simulink model "PM_fnc100a_DevHarness"  (R2022a)
settings: Solver=FixedStepDiscrete  StartTime=1  StopTime=inf  FixedStep=0.01  RelTol=1e-3
values from neighbouring files (symbols this model uses):
  rate_ms = 10    [PM_fnc1000_tc01_iter01_testsignal_builder.m]    (also in PM_fnc21_tc01_iter01_testsignal_builder.m; PM_fnc22_tc01_iter01_testsignal_builder.m)
undefined symbols (not defined in the file or in its folder): cal_abs_ampslimit_hyst_A, cal_abs_ampslimit_thresh_A, cal_cell_heat2cool_factor, cal_chg_falling_slew_rate, cal_chg_PL1_ini, cal_chg_rising_slew_rate, cal_ChgPL1_expiry_dur_thresh_ms, cal_ChgPL2_expiry_dur_thresh_ms, cal_dchg_falling_slew_rate, cal_dchg_PL1_ini, cal_dchg_rising_slew_rate, cal_DchgPL1_expiry_dur_thresh_ms, cal_DchgPL2_expiry_dur_thresh_ms, cal_table_cell_soc_percent, cal_table_cell_temp_degC, cal_table_DchgPL1_10s_limits_xtempysoc, cal_table_DchgPL1_60s_limits_xtempysoc, cal_table_DchgPL1_cont_limits_xtempysoc, cal_table_XLoad_amps_A, cal_table_XLoad_dur_ms
libraries: PM_lib x6
settings Model: PacingRate=1.600000  Creator=306427  LastModifiedBy=306427
settings SolverCC: ZeroCrossAlgorithm=Adaptive

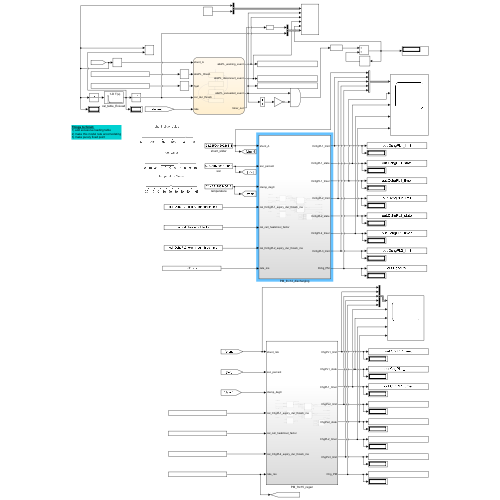
[thumbnail: Simulink's stored preview of the top-level diagram]
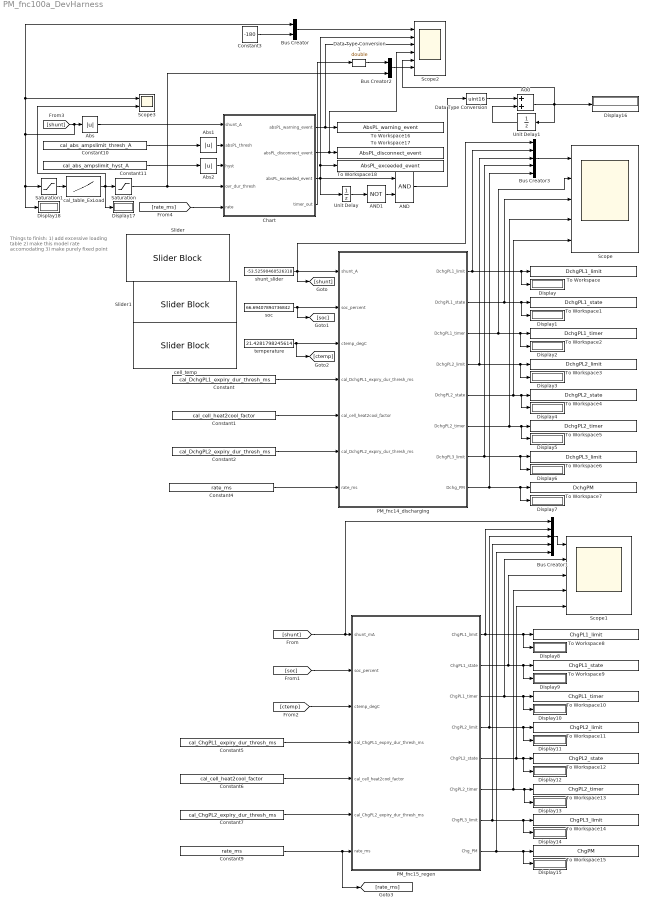
== system PM_fnc100a_DevHarness ==
  note: Things to finish:
      | 1) add excessive loading table
      | 2) make this model rate accomodating
      | 3) make purely fixed point
  AND : Logic  IconShape=distinctive  AllPortsSameDT=off  OutDataTypeStr=boolean
  AND1 : Logic  Operator=NOT  IconShape=distinctive  AllPortsSameDT=off  OutDataTypeStr=boolean
  Abs : Abs  SaturateOnIntegerOverflow=off
  Abs1 : Abs  SaturateOnIntegerOverflow=off
  Abs2 : Abs  SaturateOnIntegerOverflow=off
  Add : Sum
  Bus Creator : BusCreator  Inputs=2
  Bus Creator1 : BusCreator  Inputs=5
  Bus Creator2 : BusCreator  Inputs=2
  Bus Creator3 : BusCreator  Inputs=5
  Chart : Stateflow chart  TreatAsAtomicUnit=on
  Constant : Constant  Value=cal_DchgPL1_expiry_dur_thresh_ms
  Constant1 : Constant  Value=cal_cell_heat2cool_factor
  Constant10 : Constant  Value=cal_abs_ampslimit_thresh_A
  Constant11 : Constant  Value=cal_abs_ampslimit_hyst_A
  Constant2 : Constant  Value=cal_DchgPL2_expiry_dur_thresh_ms
  Constant3 : Constant  Value=-180
  Constant4 : Constant  Value=rate_ms
  Constant5 : Constant  Value=cal_ChgPL1_expiry_dur_thresh_ms
  Constant6 : Constant  Value=cal_cell_heat2cool_factor
  Constant7 : Constant  Value=cal_ChgPL2_expiry_dur_thresh_ms
  Constant9 : Constant  Value=rate_ms
  Data Type Conversion : DataTypeConversion  OutDataTypeStr=uint16  SaturateOnIntegerOverflow=off  RndMeth=Floor
  Data Type Conversion1 : DataTypeConversion  OutDataTypeStr=double  SaturateOnIntegerOverflow=off  RndMeth=Floor
  Display{,1..18} (19 alike) : Display
  PM_fnc14_discharging : Subsystem
  PM_fnc15_regen : Subsystem
  Saturation : Saturate  UpperLimit=3000  LowerLimit=10
  Saturation1 : Saturate  UpperLimit=2000  LowerLimit=0
  Scope : Scope  NumInputPorts=5
  Scope1 : Scope  NumInputPorts=5
  Scope2 : Scope  NumInputPorts=6
  Scope3 : Scope  NumInputPorts=2
  Slider : SliderBlock  ScaleMin=-500  ScaleMax=20
  Slider1 : SliderBlock
  To Workspace : ToWorkspace  VariableName=DchgPL1_limit  SampleTime=-1
      settings: Save2DSignal=2-D array (concatenate along first dimension)
  To Workspace1 : ToWorkspace  VariableName=DchgPL1_state  SampleTime=-1
      settings: Save2DSignal=2-D array (concatenate along first dimension)
  To Workspace10 : ToWorkspace  VariableName=ChgPL1_timer  SampleTime=-1
      settings: Save2DSignal=2-D array (concatenate along first dimension)
  To Workspace11 : ToWorkspace  VariableName=ChgPL2_limit  SampleTime=-1
      settings: Save2DSignal=2-D array (concatenate along first dimension)
  To Workspace12 : ToWorkspace  VariableName=ChgPL2_state  SampleTime=-1
      settings: Save2DSignal=2-D array (concatenate along first dimension)
  To Workspace13 : ToWorkspace  VariableName=ChgPL2_timer  SampleTime=-1
      settings: Save2DSignal=2-D array (concatenate along first dimension)
  To Workspace14 : ToWorkspace  VariableName=ChgPL3_limit  SampleTime=-1
      settings: Save2DSignal=2-D array (concatenate along first dimension)
  To Workspace15 : ToWorkspace  VariableName=ChgPM  SampleTime=-1
      settings: Save2DSignal=2-D array (concatenate along first dimension)
  To Workspace16 : ToWorkspace  VariableName=AbsPL_warning_event  SampleTime=-1
      settings: Save2DSignal=2-D array (concatenate along first dimension)
  To Workspace17 : ToWorkspace  VariableName=AbsPL_disconnect_event  SampleTime=-1
      settings: Save2DSignal=2-D array (concatenate along first dimension)
  To Workspace18 : ToWorkspace  VariableName=AbsPL_exceeded_event  SampleTime=-1
      settings: Save2DSignal=2-D array (concatenate along first dimension)
  To Workspace2 : ToWorkspace  VariableName=DchgPL1_timer  SampleTime=-1
      settings: Save2DSignal=2-D array (concatenate along first dimension)
  To Workspace3 : ToWorkspace  VariableName=DchgPL2_limit  SampleTime=-1
      settings: Save2DSignal=2-D array (concatenate along first dimension)
  To Workspace4 : ToWorkspace  VariableName=DchgPL2_state  SampleTime=-1
      settings: Save2DSignal=2-D array (concatenate along first dimension)
  To Workspace5 : ToWorkspace  VariableName=DchgPL2_timer  SampleTime=-1
      settings: Save2DSignal=2-D array (concatenate along first dimension)
  To Workspace6 : ToWorkspace  VariableName=DchgPL3_limit  SampleTime=-1
      settings: Save2DSignal=2-D array (concatenate along first dimension)
  To Workspace7 : ToWorkspace  VariableName=DchgPM  SampleTime=-1
      settings: Save2DSignal=2-D array (concatenate along first dimension)
  To Workspace8 : ToWorkspace  VariableName=ChgPL1_limit  SampleTime=-1
      settings: Save2DSignal=2-D array (concatenate along first dimension)
  To Workspace9 : ToWorkspace  VariableName=ChgPL1_state  SampleTime=-1
      settings: Save2DSignal=2-D array (concatenate along first dimension)
  Unit Delay : UnitDelay  SampleTime=-1  HasFrameUpgradeWarning=on
  Unit Delay1 : UnitDelay  SampleTime=-1  HasFrameUpgradeWarning=on
  cal_table_ExLoad : Lookup_n-D  NumberOfTableDimensions=1  BreakpointsForDimension1=cal_table_XLoad_amps_A  BeginIndexSearchUsingPreviousIndexResult=on  Table=cal_table_XLoad_dur_ms  ExtrapMethod=Clip  UseLastTableValue=on  InternalRulePriority=Speed  RndMeth=Simplest
  cell_temp : SliderBlock  ScaleMin=-20  ScaleMax=65
  shunt_slider : Constant  Value=-53.52590460526318  OutDataTypeStr=double
  soc : Constant  Value=66.69407894736842  OutDataTypeStr=double
  temperature : Constant  Value=21.4281798245614  OutDataTypeStr=double
  wires:
  soc/1 -> PM_fnc14_discharging/2(soc_percent), [soc]
  temperature/1 -> [ctemp], PM_fnc14_discharging/3(ctemp_degC)
  PM_fnc14_discharging/2(DchgPL1_state) -> Display1/1, To Workspace1/1, Scope/3
  PM_fnc14_discharging/3(DchgPL1_timer) -> To Workspace2/1, Display2/1, Scope/2
  PM_fnc14_discharging/5(DchgPL2_state) -> Display4/1, To Workspace4/1, Scope/5
  Bus Creator3/1 -> Scope/1
  PM_fnc14_discharging/6(DchgPL2_timer) -> Display5/1, To Workspace5/1, Scope/4
  PM_fnc15_regen/6(ChgPL2_timer) -> To Workspace13/1, Display13/1, Scope1/4
  PM_fnc15_regen/3(ChgPL1_timer) -> To Workspace10/1, Display10/1, Scope1/2
  PM_fnc15_regen/5(ChgPL2_state) -> To Workspace12/1, Display12/1, Scope1/5
  [shunt] -> Bus Creator1/1, PM_fnc15_regen/1(shunt_mA)
  [ctemp] -> PM_fnc15_regen/3(ctemp_degC)
  [soc] -> PM_fnc15_regen/2(soc_percent)
  Bus Creator1/1 -> Scope1/1
  PM_fnc15_regen/2(ChgPL1_state) -> To Workspace9/1, Display9/1, Scope1/3
  [shunt] -> Bus Creator/1, Scope3/1, Display18/1, Saturation1/1, Abs/1
  Abs1/1 -> Chart/2(absPL_thresh)
  Abs/1 -> Chart/1(shunt_A)
  Abs2/1 -> Chart/3(hyst)
  Chart/1(absPL_warning_event) -> To Workspace16/1, Scope2/3
  Chart/2(absPL_disconnect_event) -> To Workspace17/1, Scope2/4
  Unit Delay/1 -> AND1/1
  AND1/1 -> AND/2
  Add/1 -> Scope2/5, Display16/1, Unit Delay1/1
  AND/1 -> Data Type Conversion/1
  Unit Delay1/1 -> Add/2
  Data Type Conversion/1 -> Add/1
  cal_table_ExLoad/1 -> Scope3/2, Display17/1, Saturation/1
  [rate_ms] -> Chart/5(rate)
  Saturation/1 -> Bus Creator2/2, Chart/4(ovr_dur_thresh)
  Saturation1/1 -> cal_table_ExLoad/1
  Constant4/1 -> PM_fnc14_discharging/7(rate_ms)
  Constant2/1 -> PM_fnc14_discharging/6(cal_DchgPL2_expiry_dur_thresh_ms)
  Constant1/1 -> PM_fnc14_discharging/5(cal_cell_heat2cool_factor)
  Constant/1 -> PM_fnc14_discharging/4(cal_DchgPL1_expiry_dur_thresh_ms)
  Constant10/1 -> Abs1/1
  Constant11/1 -> Abs2/1
  Constant6/1 -> PM_fnc15_regen/5(cal_cell_heat2cool_factor)
  Constant9/1 -> [rate_ms], PM_fnc15_regen/7(rate_ms)
  Constant5/1 -> PM_fnc15_regen/4(cal_ChgPL1_expiry_dur_thresh_ms)
  Constant7/1 -> PM_fnc15_regen/6(cal_ChgPL2_expiry_dur_thresh_ms)
  PM_fnc15_regen/1(ChgPL1_limit) -> Bus Creator1/2, To Workspace8/1, Display8/1
  PM_fnc15_regen/4(ChgPL2_limit) -> Bus Creator1/3, To Workspace11/1, Display11/1
  PM_fnc15_regen/8(Chg_PM) -> Bus Creator1/5, Display15/1, To Workspace15/1
  PM_fnc15_regen/7(ChgPL3_limit) -> Bus Creator1/4, To Workspace14/1, Display14/1
  shunt_slider/1 -> Bus Creator3/1, PM_fnc14_discharging/1(shunt_A), [shunt]
  PM_fnc14_discharging/1(DchgPL1_limit) -> Bus Creator3/2, Display/1, To Workspace/1
  PM_fnc14_discharging/8(Dchg_PM) -> Bus Creator3/5, Display7/1, To Workspace7/1
  PM_fnc14_discharging/7(DchgPL3_limit) -> Bus Creator3/4, Display6/1, To Workspace6/1
  PM_fnc14_discharging/4(DchgPL2_limit) -> Bus Creator3/3, To Workspace3/1, Display3/1
  Bus Creator/1 -> Scope2/1
  Constant3/1 -> Bus Creator/2
  Chart/4(timer_out) -> Data Type Conversion1/1
  Chart/3(absPL_exceeded_event) -> Scope2/2, To Workspace18/1, Unit Delay/1, AND/1
  Bus Creator2/1 -> Scope2/6
  Data Type Conversion1/1 -> Bus Creator2/1

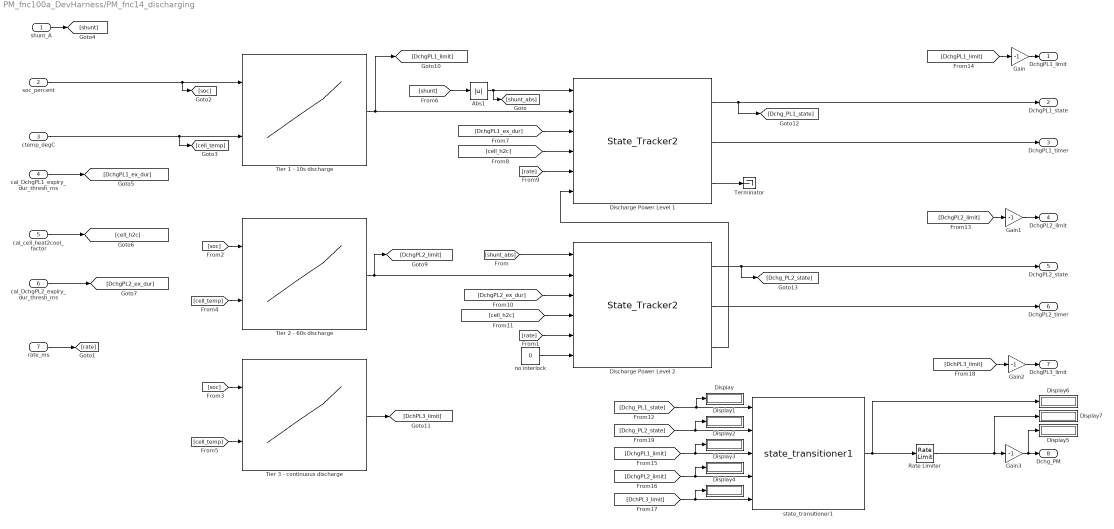
== system PM_fnc100a_DevHarness/PM_fnc14_discharging ==
  shunt_A : Inport
  soc_percent : Inport  Port=2
  ctemp_degC : Inport  Port=3
  cal_DchgPL1_expiry_dur_thresh_ms : Inport  Port=4
  cal_cell_heat2cool_factor : Inport  Port=5
  cal_DchgPL2_expiry_dur_thresh_ms : Inport  Port=6
  rate_ms : Inport  Port=7
  Abs1 : Abs  SaturateOnIntegerOverflow=off
  Discharge Power Level 1 : PM_lib/State_Tracker2  SystemSampleTime=-1  VariantActivationTime=update diagram  Latency=0  AutoFrameSizeCalculation=off
  Discharge Power Level 2 : PM_lib/State_Tracker2  SystemSampleTime=-1  VariantActivationTime=update diagram  Latency=0  AutoFrameSizeCalculation=off
  Display{,1..7} (8 alike) : Display
  Gain : Gain  Gain=-1  ParamDataTypeStr=int8  OutDataTypeStr=Inherit: Same as input
  Gain1 : Gain  Gain=-1  ParamDataTypeStr=int8  OutDataTypeStr=Inherit: Same as input
  Gain2 : Gain  Gain=-1  ParamDataTypeStr=int8  OutDataTypeStr=Inherit: Same as input
  Gain3 : Gain  Gain=-1  ParamDataTypeStr=int8
  Rate Limiter : RateLimiter  RisingSlewLimit=cal_dchg_rising_slew_rate  FallingSlewLimit=cal_dchg_falling_slew_rate  SampleTimeMode=inherited  InitialCondition=cal_dchg_PL1_ini
  Terminator : Terminator
  Tier 1 - 10s discharge : Lookup_n-D  BreakpointsForDimension1=cal_table_cell_soc_percent  BreakpointsForDimension2=cal_table_cell_temp_degC  BeginIndexSearchUsingPreviousIndexResult=on  Table=cal_table_DchgPL1_10s_limits_xtempysoc  ExtrapMethod=Clip  UseLastTableValue=on  InternalRulePriority=Speed  OutDataTypeStr=double  RndMeth=Simplest  InputSameDT=off
      settings: InputPortMap=u0,u1
  Tier 2 - 60s discharge : Lookup_n-D  BreakpointsForDimension1=cal_table_cell_soc_percent  BreakpointsForDimension2=cal_table_cell_temp_degC  BeginIndexSearchUsingPreviousIndexResult=on  Table=cal_table_DchgPL1_60s_limits_xtempysoc  ExtrapMethod=Clip  UseLastTableValue=on  InternalRulePriority=Speed  OutDataTypeStr=double  RndMeth=Simplest  InputSameDT=off
      settings: InputPortMap=u0,u1
  Tier 3 - continuous discharge : Lookup_n-D  BreakpointsForDimension1=cal_table_cell_soc_percent  BreakpointsForDimension2=cal_table_cell_temp_degC  BeginIndexSearchUsingPreviousIndexResult=on  Table=cal_table_DchgPL1_cont_limits_xtempysoc  ExtrapMethod=Clip  UseLastTableValue=on  InternalRulePriority=Speed  OutDataTypeStr=double  RndMeth=Simplest  InputSameDT=off
      settings: InputPortMap=u0,u1
  no interlock : Constant  Value=0  OutDataTypeStr=boolean
  state_transitioner1 : PM_lib/state_transitioner1  SystemSampleTime=-1  VariantActivationTime=update diagram  Latency=0  AutoFrameSizeCalculation=off
  DchgPL1_limit : Outport
  DchgPL1_state : Outport  Port=2
  DchgPL1_timer : Outport  Port=3
  DchgPL2_limit : Outport  Port=4
  DchgPL2_state : Outport  Port=5
  DchgPL2_timer : Outport  Port=6
  DchgPL3_limit : Outport  Port=7
  Dchg_PM : Outport  Port=8
  wires:
  [cell_temp] -> Tier 3 - continuous discharge/2
  Discharge Power Level 2/2 -> DchgPL2_timer/1
  [soc] -> Tier 2 - 60s discharge/1
  [cell_temp] -> Tier 2 - 60s discharge/2
  ctemp_degC/1 -> [cell_temp], Tier 1 - 10s discharge/2
  cal_DchgPL2_expiry_dur_thresh_ms/1 -> [DchgPL2_ex_dur]
  Tier 2 - 60s discharge/1 -> [DchgPL2_limit], Discharge Power Level 2/2
  Discharge Power Level 2/1 -> DchgPL2_state/1, [Dchg_PL2_state]
  Discharge Power Level 1/2 -> DchgPL1_timer/1
  Discharge Power Level 1/1 -> DchgPL1_state/1, [Dchg_PL1_state]
  [rate] -> Discharge Power Level 2/5
  [soc] -> Tier 3 - continuous discharge/1
  rate_ms/1 -> [rate]
  cal_DchgPL1_expiry_dur_thresh_ms/1 -> [DchgPL1_ex_dur]
  [shunt_abs] -> Discharge Power Level 2/1
  Abs1/1 -> Discharge Power Level 1/1, [shunt_abs]
  shunt_A/1 -> [shunt]
  cal_cell_heat2cool_factor/1 -> [cell_h2c]
  Tier 1 - 10s discharge/1 -> Discharge Power Level 1/2, [DchgPL1_limit]
  soc_percent/1 -> [soc], Tier 1 - 10s discharge/1
  [shunt] -> Abs1/1
  [DchgPL2_ex_dur] -> Discharge Power Level 2/3
  [rate] -> Discharge Power Level 1/5
  [DchgPL1_ex_dur] -> Discharge Power Level 1/3
  no interlock/1 -> Discharge Power Level 2/6
  Discharge Power Level 2/3 -> Discharge Power Level 1/6
  Discharge Power Level 1/3 -> Terminator/1
  [DchgPL2_limit] -> Gain1/1
  [DchgPL1_limit] -> Gain/1
  [DchgPL1_limit] -> Display2/1, state_transitioner1/3
  [DchgPL2_limit] -> Display3/1, state_transitioner1/4
  Tier 3 - continuous discharge/1 -> [DchPL3_limit]
  [DchPL3_limit] -> Display4/1, state_transitioner1/5
  [DchPL3_limit] -> Gain2/1
  Gain/1 -> DchgPL1_limit/1
  Gain1/1 -> DchgPL2_limit/1
  Gain2/1 -> DchgPL3_limit/1
  Gain3/1 -> Display5/1, Dchg_PM/1
  [Dchg_PL1_state] -> Display/1, state_transitioner1/1
  [Dchg_PL2_state] -> Display1/1, state_transitioner1/2
  [cell_h2c] -> Discharge Power Level 1/4
  [cell_h2c] -> Discharge Power Level 2/4
  state_transitioner1/1 -> Rate Limiter/1, Display6/1
  Rate Limiter/1 -> Display7/1, Gain3/1

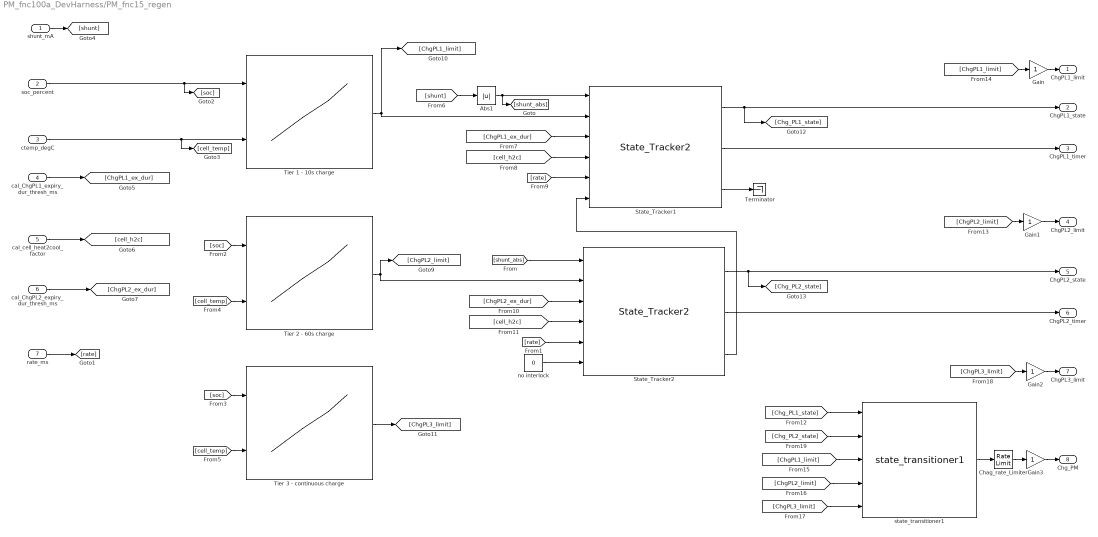
== system PM_fnc100a_DevHarness/PM_fnc15_regen ==
  shunt_mA : Inport
  soc_percent : Inport  Port=2
  ctemp_degC : Inport  Port=3
  cal_ChgPL1_expiry_dur_thresh_ms : Inport  Port=4
  cal_cell_heat2cool_factor : Inport  Port=5
  cal_ChgPL2_expiry_dur_thresh_ms : Inport  Port=6
  rate_ms : Inport  Port=7
  Abs1 : Abs  SaturateOnIntegerOverflow=off
  Chag_rate_Limiter : RateLimiter  RisingSlewLimit=cal_chg_rising_slew_rate  FallingSlewLimit=cal_chg_falling_slew_rate  SampleTimeMode=inherited  InitialCondition=cal_chg_PL1_ini
  Gain : Gain  OutDataTypeStr=Inherit: Same as input
  Gain1 : Gain  ParamDataTypeStr=Inherit: Same as input
  Gain2 : Gain  ParamDataTypeStr=Inherit: Same as input
  Gain3 : Gain  ParamDataTypeStr=Inherit: Same as input
  State_Tracker1 : PM_lib/State_Tracker2  SystemSampleTime=-1  VariantActivationTime=update diagram  Latency=0  AutoFrameSizeCalculation=off
  State_Tracker2 : PM_lib/State_Tracker2  SystemSampleTime=-1  VariantActivationTime=update diagram  Latency=0  AutoFrameSizeCalculation=off
  Terminator : Terminator
  Tier 1 - 10s charge : Lookup_n-D  BreakpointsForDimension1=cal_table_cell_soc_percent  BreakpointsForDimension2=cal_table_cell_temp_degC  BeginIndexSearchUsingPreviousIndexResult=on  Table=cal_table_DchgPL1_10s_limits_xtempysoc  ExtrapMethod=Clip  UseLastTableValue=on  InternalRulePriority=Speed  RndMeth=Simplest  InputSameDT=off
      settings: InputPortMap=u0,u1
  Tier 2 - 60s charge : Lookup_n-D  BreakpointsForDimension1=cal_table_cell_soc_percent  BreakpointsForDimension2=cal_table_cell_temp_degC  BeginIndexSearchUsingPreviousIndexResult=on  Table=cal_table_DchgPL1_60s_limits_xtempysoc  ExtrapMethod=Clip  UseLastTableValue=on  InternalRulePriority=Speed  RndMeth=Simplest  InputSameDT=off
      settings: InputPortMap=u0,u1
  Tier 3 - continuous charge : Lookup_n-D  BreakpointsForDimension1=cal_table_cell_soc_percent  BreakpointsForDimension2=cal_table_cell_temp_degC  BeginIndexSearchUsingPreviousIndexResult=on  Table=cal_table_DchgPL1_cont_limits_xtempysoc  ExtrapMethod=Clip  UseLastTableValue=on  InternalRulePriority=Speed  RndMeth=Simplest  InputSameDT=off
      settings: InputPortMap=u0,u1
  no interlock : Constant  Value=0  OutDataTypeStr=boolean
  state_transitioner1 : PM_lib/state_transitioner1  SystemSampleTime=-1  VariantActivationTime=update diagram  Latency=0  AutoFrameSizeCalculation=off
  ChgPL1_limit : Outport
  ChgPL1_state : Outport  Port=2
  ChgPL1_timer : Outport  Port=3
  ChgPL2_limit : Outport  Port=4
  ChgPL2_state : Outport  Port=5
  ChgPL2_timer : Outport  Port=6
  ChgPL3_limit : Outport  Port=7
  Chg_PM : Outport  Port=8
  wires:
  [cell_temp] -> Tier 3 - continuous charge/2
  State_Tracker2/2 -> ChgPL2_timer/1
  [soc] -> Tier 2 - 60s charge/1
  [cell_temp] -> Tier 2 - 60s charge/2
  ctemp_degC/1 -> [cell_temp], Tier 1 - 10s charge/2
  [rate] -> State_Tracker1/5
  cal_ChgPL2_expiry_dur_thresh_ms/1 -> [ChgPL2_ex_dur]
  Tier 2 - 60s charge/1 -> State_Tracker2/2, [ChgPL2_limit]
  State_Tracker2/1 -> ChgPL2_state/1, [Chg_PL2_state]
  State_Tracker1/2 -> ChgPL1_timer/1
  State_Tracker1/1 -> ChgPL1_state/1, [Chg_PL1_state]
  [rate] -> State_Tracker2/5
  [soc] -> Tier 3 - continuous charge/1
  rate_ms/1 -> [rate]
  cal_ChgPL1_expiry_dur_thresh_ms/1 -> [ChgPL1_ex_dur]
  [shunt_abs] -> State_Tracker2/1
  Abs1/1 -> State_Tracker1/1, [shunt_abs]
  shunt_mA/1 -> [shunt]
  cal_cell_heat2cool_factor/1 -> [cell_h2c]
  Tier 1 - 10s charge/1 -> State_Tracker1/2, [ChgPL1_limit]
  soc_percent/1 -> [soc], Tier 1 - 10s charge/1
  [shunt] -> Abs1/1
  [ChgPL2_ex_dur] -> State_Tracker2/3
  [ChgPL1_ex_dur] -> State_Tracker1/3
  no interlock/1 -> State_Tracker2/6
  State_Tracker2/3 -> State_Tracker1/6
  State_Tracker1/3 -> Terminator/1
  state_transitioner1/1 -> Chag_rate_Limiter/1
  [ChgPL2_limit] -> Gain1/1
  [ChgPL1_limit] -> Gain/1
  [ChgPL1_limit] -> state_transitioner1/3
  [ChgPL2_limit] -> state_transitioner1/4
  Tier 3 - continuous charge/1 -> [ChgPL3_limit]
  [ChgPL3_limit] -> state_transitioner1/5
  [ChgPL3_limit] -> Gain2/1
  Gain/1 -> ChgPL1_limit/1
  Gain1/1 -> ChgPL2_limit/1
  Gain2/1 -> ChgPL3_limit/1
  Gain3/1 -> Chg_PM/1
  Chag_rate_Limiter/1 -> Gain3/1
  [Chg_PL1_state] -> state_transitioner1/1
  [Chg_PL2_state] -> state_transitioner1/2
  [cell_h2c] -> State_Tracker1/4
  [cell_h2c] -> State_Tracker2/4

== stateflow chart PM_fnc100a_DevHarness/Chart ==
  state RESET
    timer = 0;
    absPL_exceeded_event = boolean(0);
    absPL_warning_event = boolean(0);
    absPL_disconnect_event = boolean(0);
  state MEAS_DURATION
    timer = timer + rate;
    timer_out = timer;
    absPL_exceeded_event = boolean(1);
    absPL_warning_event = boolean(0);
    absPL_disconnect_event = boolean(0);
  state WARNING
    timer = timer + rate;
    timer_out = timer;
    absPL_warning_event = boolean(1);
    absPL_disconnect_event = boolean(0);
  state DISCONNECT
    timer = timer + rate;
    timer_out = timer;
    absPL_disconnect_event = boolean(1);
  (default) -> RESET
  WARNING -> RESET [order 1] : [shunt_A < absPL_thresh - hyst]
  RESET -> MEAS_DURATION : [shunt_A > absPL_thresh]
  MEAS_DURATION -> RESET [order 2] : [shunt_A < absPL_thresh -hyst]
  MEAS_DURATION -> DISCONNECT [order 3] : [timer > ovr_dur_thresh]
  MEAS_DURATION -> WARNING [order 1] : [timer >= 1000]
  WARNING -> DISCONNECT [order 3] : [timer > ovr_dur_thresh]
  WARNING -> DISCONNECT [order 2] : [timer > 3000]
  data: timer local uint16; absPL_warning_event output; absPL_disconnect_event output; shunt_A input; absPL_thresh input; hyst input; ovr_dur_thresh input; rate input; absPL_exceeded_event output; timer_out output
